simulink model "AprilTagHIL"  (R2024b)
settings: Solver=ode4  StartTime=0.0  StopTime=Tsim  FixedStep=0.005  RelTol=1e-3
values from neighbouring files (symbols this model uses):
  Caf = 20    [AprilTagHILSetup.m]
  Car = 20    [AprilTagHILSetup.m]
  circle_dir = 1    [AprilTagHILSetup.m]
  delta_corr_max_rad = deg2rad(8)    [AprilTagHILSetup.m]
  delta_max_rad = deg2rad(25)    [AprilTagHILSetup.m]
  delta_test_rad = deg2rad(14.6)    [AprilTagHILSetup.m]
  dist_psi_down_time_s = 10.0    (= 10)    [AprilTagHILSetup.m]
  dist_psi_step_amp_rad = deg2rad(10)    [AprilTagHILSetup.m]
  dist_psi_up_time_s = 9.0    (= 9)    [AprilTagHILSetup.m]
  dist_x_down_time_s = 6.0    (= 6)    [AprilTagHILSetup.m]
  dist_x_step_amp_m = 0.10    (= 0.1)    [AprilTagHILSetup.m]
  dist_x_up_time_s = 5.0    (= 5)    [AprilTagHILSetup.m]
  dist_y_down_time_s = 8.0    (= 8)    [AprilTagHILSetup.m]
  dist_y_up_time_s = 7.0    (= 7)    [AprilTagHILSetup.m]
  Jz = 0.015    [AprilTagHILSetup.m]
  K_psi = 0.8    [AprilTagHILSetup.m]
  K_r = 0.05    [AprilTagHILSetup.m]
  K_radius = 0.4    [AprilTagHILSetup.m]
  Kd_psi_pid = 0.0    (= 0)    [AprilTagHILSetup.m]
  Kd_radius_pid = 0.0    (= 0)    [AprilTagHILSetup.m]
  Ki_psi_pid = 0.0    (= 0)    [AprilTagHILSetup.m]
  Ki_radius_pid = 0.0    (= 0)    [AprilTagHILSetup.m]
  Kp_psi_pid = 1.0    (= 1)    [AprilTagHILSetup.m]
  Kp_radius_pid = 0.65    [AprilTagHILSetup.m]
  L = 0.26    [AprilTagHILSetup.m]
  lf = 0.13    [AprilTagHILSetup.m]
  lr = 0.13    [AprilTagHILSetup.m]
  m = 1.5    [AprilTagHILSetup.m]
  noise_psi_std_rad = deg2rad(0.5)    [AprilTagHILSetup.m]
  noise_x_std_m = 0.005    [AprilTagHILSetup.m]
  noise_y_std_m = 0.005    [AprilTagHILSetup.m]
  psi0_rad = pi/2 - deg2rad(45)    [AprilTagHILSetup.m]
  psi_offset_max_rad = deg2rad(18)    [AprilTagHILSetup.m]
  r0_radps = 0.0    (= 0)    [AprilTagHILSetup.m]
  R_ref = 1.0    (= 1)    [AprilTagHILSetup.m]
  Ts_vision = 0.05    [AprilTagHILSetup.m]
  Vx_const = 1.0    (= 1)    [AprilTagHILSetup.m]
  Vy0 = 0.0    (= 0)    [AprilTagHILSetup.m]
  X0 = 0.4    [AprilTagHILSetup.m]
  xc = 0.0    (= 0)    [AprilTagHILSetup.m]
  Y0 = 0.0    (= 0)    [AprilTagHILSetup.m]
  yc = 0.0    (= 0)    [AprilTagHILSetup.m]
libraries: slpidlib x2
settings Model: Creator=mateu  LastModifiedBy=mateu

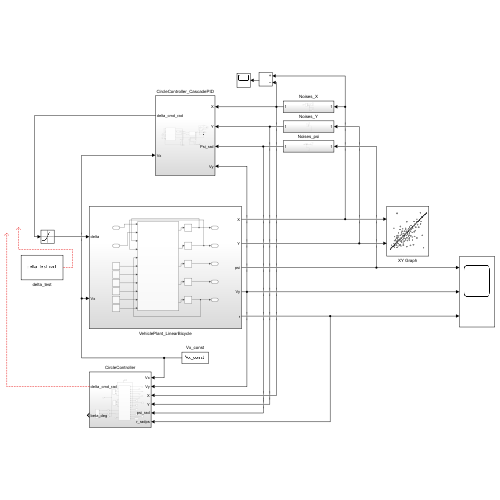
[thumbnail: Simulink's stored preview of the top-level diagram]
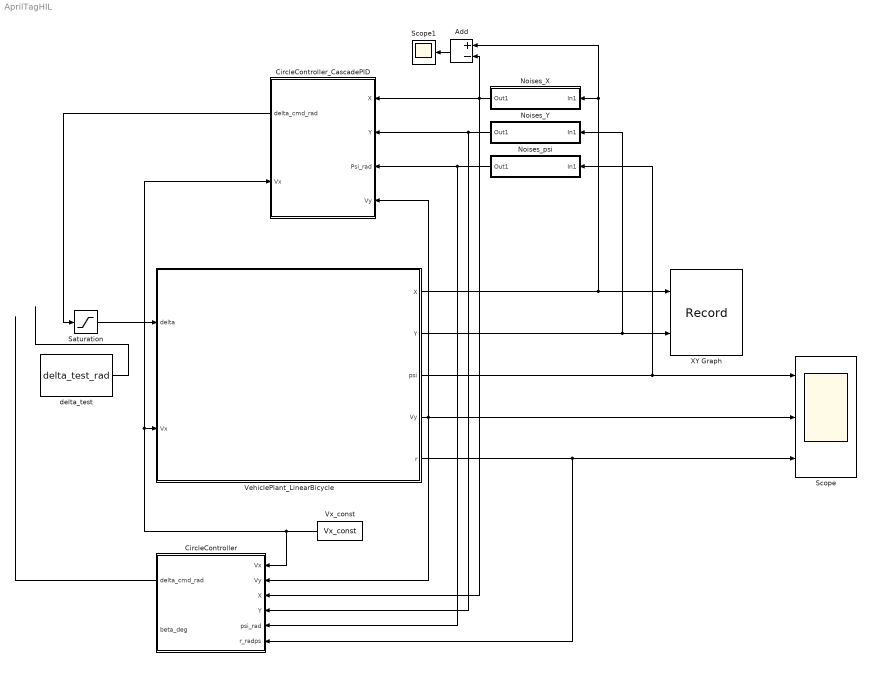
== system AprilTagHIL ==
  Add : Sum  Inputs=+-
  CircleController : Subsystem
  CircleController_CascadePID : Subsystem
      settings: PortSchema="{\"entries\":[{\"content\":{\"sides\":[{\"content\":{\"connectorIds\":[\"In1\",\"In2\",\"In3\",\"In4\"]},\"type\":\"ConnectorPlacement.EquallySpacedRectSide\",\"uuid\":\"4ebb86b3-f174-446a-9526-2905becb2528\"},{\"content\":{\"connectorIds\":[\"Out1\",\"In5\"],\"side\":\"RIGHT\"},\"type\":\"ConnectorPlacement.EquallySpacedRectSide\",\"uuid\":\"60998215-3f76-4645-a7df-e26e298f7453\"},{\"content\":{\"side\":\"TOP\"},\"type\":\"ConnectorPlacement.EquallySpacedRectSide\",\"uuid\":\"c14afc2e-0d09-4288-83d9-90a5a30cc5d5\"}]},\"type\":\"ConnectorPlacement.EquallySpacedConnector\",\"uuid\":\"bc3aa7c0-8848-4f28-b7fa-9a6d41e7c366\"}],\"packageUris\":[\"http://schema.mathworks.com/mf0/Connector/R2020b\"],\"version\":\"1.0\"}"
  Noises_X : Subsystem
  Noises_Y : Subsystem
  Noises_psi : Subsystem
  Saturation : Saturate  UpperLimit=delta_max_rad  LowerLimit=-delta_max_rad
  Scope : Scope  NumInputPorts=3
  Scope1 : Scope
  VehiclePlant_LinearBicycle : Subsystem
  Vx_const : Constant  Value=Vx_const
  XY Graph : Record  FileSettingsInternal="{\"entries\":[{\"content\":{\"excelSettings\":{\"content\":{},\"type\":\"Streamout.ExcelSettings\"}},\"type\":\"Streamout.FileSettingStorage\",\"uuid\":\"\"}],\"packageUris\":[\"http:\\/\\/schema.mathworks.com\\/mf0\\/streamout_blocks\\/R2020a\"],\"version\":\"1.0\"}"  Layout=[1 1]  SignalsInternal="{\"entries\":[{\"content\":{\"signals\":[{\"content\":{\"blockPath\":[],\"dimensions\":[1],\"domain\":\"\",\"lineColor\":\"#a2142f\",\"plots\":[ 1 ],\"port\":1,\"sid\":[\"\"],\"signalID\":1,\"signalName\":\"VehiclePlant_LinearBicycle:1\"},\"type\":\"RecordBlkView.Signal\",\"uuid\":\"\"},{\"content\":{\"blockPath\":[],\"dimensions\":[1],\"domain\":\"\",\"lineColor\":\"#139fff\",\"plots\":[ 1 ],\"port\":2,\"sid\":[\"\"],\"signalID\":2,\"signalName\":\"VehiclePlant_LinearBicycle:2\"},\"type\":\"RecordBlkView.Signal\",\"uuid\":\"\"}]},\"type\":\"RecordBlkView.InputSignals\",\"uuid\":\"\"}],\"packageUris\":[\"http:\\/\\/schema.mathworks.com\\/mf0\\/streamout_blocks\\/R2020a\"],\"version\":\"1.0\"}"  VisualizationBindings="{\"xyplotplugin\":{\"info\":[{\"series\":[{\"bindingParametersList\":[{\"parameter\":\"X-Axis\",\"signalID\":1,\"signalName\":\"VehiclePlant_LinearBicycle:1\"},{\"parameter\":\"Y-Axis\",\"signalID\":2,\"signalName\":\"VehiclePlant_LinearBicycle:2\"}],\"seriesID\":0}],\"subplotID\":1}]}}"  CompatibilityTag=XY
  delta_test : Constant  Value=delta_test_rad
  wires:
  Vx_const/1 -> CircleController/1(Vx), CircleController_CascadePID/5(Vx), VehiclePlant_LinearBicycle/2(Vx)
  Saturation/1 -> VehiclePlant_LinearBicycle/1(delta)
  VehiclePlant_LinearBicycle/1(X) -> XY Graph/1, Add/1, Noises_X/1(In1)
  VehiclePlant_LinearBicycle/4(Vy) -> CircleController_CascadePID/4(Vy), Scope/2, CircleController/2(Vy)
  VehiclePlant_LinearBicycle/5(r) -> Scope/3, CircleController/6(r_radps)
  VehiclePlant_LinearBicycle/3(psi) -> Noises_psi/1(In1), Scope/1
  VehiclePlant_LinearBicycle/2(Y) -> XY Graph/2, Noises_Y/1(In1)
  CircleController_CascadePID/1(delta_cmd_rad) -> Saturation/1
  Noises_Y/1(Out1) -> CircleController_CascadePID/2(Y), CircleController/4(Y)
  Noises_X/1(Out1) -> Add/2, CircleController_CascadePID/1(X), CircleController/3(X)
  Noises_psi/1(Out1) -> CircleController_CascadePID/3(Psi_rad), CircleController/5(psi_rad)
  Add/1 -> Scope1/1
  CircleController/1(delta_cmd_rad) -> ?
  delta_test/1 -> ?

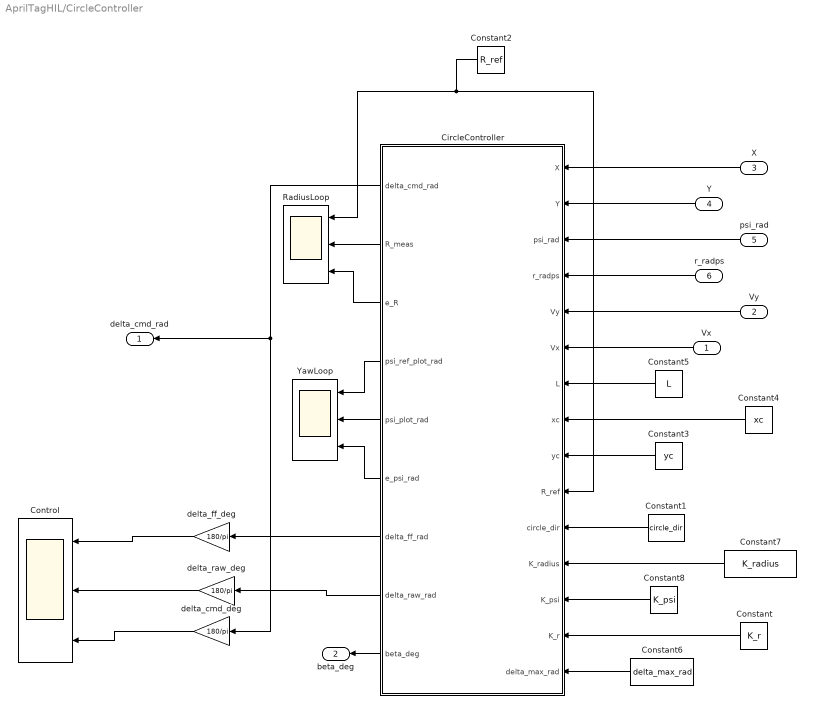
== system AprilTagHIL/CircleController ==
  Vx : Inport
  Vy : Inport  Port=2
  X : Inport  Port=3
  Y : Inport  Port=4
  psi_rad : Inport  Port=5
  r_radps : Inport  Port=6
  CircleController : MATLAB Function  TreatAsAtomicUnit=on
  Constant : Constant  Value=K_r
  Constant1 : Constant  Value=circle_dir
  Constant2 : Constant  Value=R_ref
  Constant3 : Constant  Value=yc
  Constant4 : Constant  Value=xc
  Constant5 : Constant  Value=L
  Constant6 : Constant  Value=delta_max_rad
  Constant7 : Constant  Value=K_radius
  Constant8 : Constant  Value=K_psi
  Control : Scope  NumInputPorts=3
  RadiusLoop : Scope  NumInputPorts=3
  YawLoop : Scope  NumInputPorts=3
  delta_cmd_deg : Gain  Gain=180/pi
  delta_ff_deg : Gain  Gain=180/pi
  delta_raw_deg : Gain  Gain=180/pi
  delta_cmd_rad : Outport
  beta_deg : Outport  Port=2
  wires:
  Vx/1 -> CircleController/6(Vx)
  CircleController/3(e_R) -> RadiusLoop/3
  CircleController/5(psi_plot_rad) -> YawLoop/2
  Constant1/1 -> CircleController/11(circle_dir)
  CircleController/7(delta_ff_rad) -> delta_ff_deg/1
  CircleController/9(beta_deg) -> beta_deg/1
  CircleController/4(psi_ref_plot_rad) -> YawLoop/1
  CircleController/6(e_psi_rad) -> YawLoop/3
  CircleController/8(delta_raw_rad) -> delta_raw_deg/1
  CircleController/2(R_meas) -> RadiusLoop/2
  CircleController/1(delta_cmd_rad) -> delta_cmd_deg/1, delta_cmd_rad/1
  Constant/1 -> CircleController/14(K_r)
  Constant4/1 -> CircleController/8(xc)
  X/1 -> CircleController/1(X)
  Constant3/1 -> CircleController/9(yc)
  Y/1 -> CircleController/2(Y)
  psi_rad/1 -> CircleController/3(psi_rad)
  r_radps/1 -> CircleController/4(r_radps)
  delta_raw_deg/1 -> Control/2
  Vy/1 -> CircleController/5(Vy)
  Constant5/1 -> CircleController/7(L)
  Constant7/1 -> CircleController/12(K_radius)
  Constant8/1 -> CircleController/13(K_psi)
  Constant6/1 -> CircleController/15(delta_max_rad)
  delta_ff_deg/1 -> Control/1
  delta_cmd_deg/1 -> Control/3
  Constant2/1 -> RadiusLoop/1, CircleController/10(R_ref)

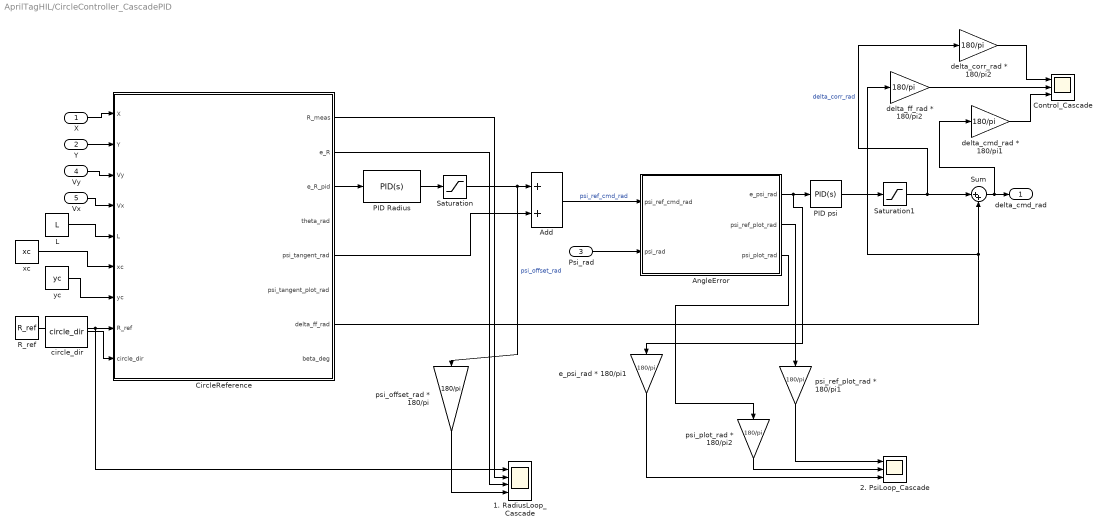
== system AprilTagHIL/CircleController_CascadePID ==
  X : Inport
  Y : Inport  Port=2
  Psi_rad : Inport  Port=3
  Vy : Inport  Port=4
  Vx : Inport  Port=5
  1. RadiusLoop_Cascade : Scope  NumInputPorts=4
  2. PsiLoop_Cascade : Scope  NumInputPorts=3
  Add : Sum
  AngleError : MATLAB Function  TreatAsAtomicUnit=on
  CircleReference : MATLAB Function  TreatAsAtomicUnit=on
  Control_Cascade : Scope  NumInputPorts=3
  L : Constant  Value=L
  PID Radius : slpidlib/PID Controller  Controller=PID  Form=Parallel  TimeDomain=Continuous-time  UseExternalTs=off  SampleTime=-1  IntegratorMethod=Forward Euler  FilterMethod=Forward Euler  ControllerParametersSource=internal  P=Kp_radius_pid  I=Ki_radius_pid  UseKiTs=off  D=Kd_radius_pid  UseExternalDerivativeSource=off  N=171.856773592637  UseFilter=on  TunerSelectOption=Transfer Function Based (PID Tuner App)  InitialConditionSource=internal  InitialConditionForIntegrator=0  InitialConditionForFilter=0  DifferentiatorICPrevScaledInput=0  ExternalReset=none  TrackingMode=off  Kt=1  LimitOutput=off  SatLimitsSource=internal  UpperSaturationLimit=inf  LowerSaturationLimit=-inf  LinearizeAsGain=on  AntiWindupMode=none  Kb=1  LimitIntegrator=off  UpperIntegratorSaturationLimit=inf  LowerIntegratorSaturationLimit=-inf  POutMin=[]  POutMax=[]  IOutMin=[]  IOutMax=[]  DOutMin=[]  DOutMax=[]  NOutMin=[]  NOutMax=[]  SumOutMin=[]  SumOutMax=[]  SaturationOutMin=[]  SaturationOutMax=[]  PParamMin=[]  PParamMax=[]  IParamMin=[]  IParamMax=[]  DParamMin=[]  DParamMax=[]  NParamMin=[]  NParamMax=[]  KbParamMin=[]  KbParamMax=[]  KtParamMin=[]  KtParamMax=[]  KbOutMin=[]  KbOutMax=[]  KtOutMin=[]  KtOutMax=[]  IntegratorOutMin=[]  IntegratorOutMax=[]  FilterOutMin=[]  FilterOutMax=[]  SumI1OutMin=[]  SumI1OutMax=[]  SumI2OutMin=[]  SumI2OutMax=[]  SumI3OutMin=[]  SumI3OutMax=[]  SumI4OutMin=[]  SumI4OutMax=[]  SumDOutMin=[]  SumDOutMax=[]  DifferentiatorOutMin=[]  DifferentiatorOutMax=[]  FilterDiffOutCoefMin=[]  FilterDiffOutCoefMax=[]  ReciprocalOutMin=[]  ReciprocalOutMax=[]  SumDenOutMin=[]  SumDenOutMax=[]  SumNumOutMin=[]  SumNumOutMax=[]  DivideOutMin=[]  DivideOutMax=[]  UdiffTsProdOutMin=[]  UdiffTsProdOutMax=[]  NTsProdOutMin=[]  NTsProdOutMax=[]  UintegralTsProdOutMin=[]  UintegralTsProdOutMax=[]  UngainTsProdOutMin=[]  UngainTsProdOutMax=[]  ClampingZeroOutDataTypeStr=Inherit: Inherit via back propagation  ClampingZeroOutMin=[]  ClampingZeroOutMax=[]  FilterDenConstantOutDataTypeStr=Inherit: Inherit via back propagation  FilterDenConstantOutMin=[]  FilterDenConstantOutMax=[]  PCopyOutDataTypeStr=Inherit: Inherit via back propagation  PCopyOutMin=[]  PCopyOutMax=[]  NCopyOutDataTypeStr=Inherit: Inherit via back propagation  NCopyOutMin=[]  NCopyOutMax=[]  IntegratorContinuousStateAttributes=''  IntegratorStateMustResolveToSignalObject=off  IntegratorRTWStateStorageClass=Auto  FilterContinuousStateAttributes=''  FilterStateMustResolveToSignalObject=off  FilterRTWStateStorageClass=Auto  ParallelPVariant=InternalParameters  IdealPVariant=Disabled  IVariant=InternalParameters  DVariant=InternalParameters  IntegratorVariant=Continuous  SatVariant=Disabled  AWVariant=Passthrough  PCopyVariant=Disabled  TRVariant=Disabled  FdbkBlocksVariant=Forward  IdealPFdbkVariant=Disabled  SatFdbkVariant=Disabled  DerivativeFilterVariant=ContFilter  NVariant=InternalParameters  NCopyVariant=Disabled  FilterICVariant=InternalICsFilter  IntegratorICVariant=InternalICs  ExternalResetVariant=Disabled  TRSumVariant=Passthrough  SumFdbkVariant=Disabled  SumVariant=Sum_PID  TsampFilterVariant=InternalTs  TsampNgainVariant=Passthrough  TsampIntegralVariant=Disabled_SignalSpec  ExternalSaturationOutDataTypeStr=Inherit: Same as second input  DerivativeSourceVariant=ErrorSignal  PreIntVariant=InternalPreInt
  PID psi : slpidlib/PID Controller  Controller=PID  Form=Parallel  TimeDomain=Continuous-time  UseExternalTs=off  SampleTime=-1  IntegratorMethod=Forward Euler  FilterMethod=Forward Euler  ControllerParametersSource=internal  P=Kp_psi_pid  I=Ki_psi_pid  UseKiTs=off  D=Kd_psi_pid  UseExternalDerivativeSource=off  N=184.215923888363  UseFilter=on  TunerSelectOption=Transfer Function Based (PID Tuner App)  InitialConditionSource=internal  InitialConditionForIntegrator=0  InitialConditionForFilter=0  DifferentiatorICPrevScaledInput=0  ExternalReset=none  TrackingMode=off  Kt=1  LimitOutput=off  SatLimitsSource=internal  UpperSaturationLimit=inf  LowerSaturationLimit=-inf  LinearizeAsGain=on  AntiWindupMode=none  Kb=1  LimitIntegrator=off  UpperIntegratorSaturationLimit=inf  LowerIntegratorSaturationLimit=-inf  POutMin=[]  POutMax=[]  IOutMin=[]  IOutMax=[]  DOutMin=[]  DOutMax=[]  NOutMin=[]  NOutMax=[]  SumOutMin=[]  SumOutMax=[]  SaturationOutMin=[]  SaturationOutMax=[]  PParamMin=[]  PParamMax=[]  IParamMin=[]  IParamMax=[]  DParamMin=[]  DParamMax=[]  NParamMin=[]  NParamMax=[]  KbParamMin=[]  KbParamMax=[]  KtParamMin=[]  KtParamMax=[]  KbOutMin=[]  KbOutMax=[]  KtOutMin=[]  KtOutMax=[]  IntegratorOutMin=[]  IntegratorOutMax=[]  FilterOutMin=[]  FilterOutMax=[]  SumI1OutMin=[]  SumI1OutMax=[]  SumI2OutMin=[]  SumI2OutMax=[]  SumI3OutMin=[]  SumI3OutMax=[]  SumI4OutMin=[]  SumI4OutMax=[]  SumDOutMin=[]  SumDOutMax=[]  DifferentiatorOutMin=[]  DifferentiatorOutMax=[]  FilterDiffOutCoefMin=[]  FilterDiffOutCoefMax=[]  ReciprocalOutMin=[]  ReciprocalOutMax=[]  SumDenOutMin=[]  SumDenOutMax=[]  SumNumOutMin=[]  SumNumOutMax=[]  DivideOutMin=[]  DivideOutMax=[]  UdiffTsProdOutMin=[]  UdiffTsProdOutMax=[]  NTsProdOutMin=[]  NTsProdOutMax=[]  UintegralTsProdOutMin=[]  UintegralTsProdOutMax=[]  UngainTsProdOutMin=[]  UngainTsProdOutMax=[]  ClampingZeroOutDataTypeStr=Inherit: Inherit via back propagation  ClampingZeroOutMin=[]  ClampingZeroOutMax=[]  FilterDenConstantOutDataTypeStr=Inherit: Inherit via back propagation  FilterDenConstantOutMin=[]  FilterDenConstantOutMax=[]  PCopyOutDataTypeStr=Inherit: Inherit via back propagation  PCopyOutMin=[]  PCopyOutMax=[]  NCopyOutDataTypeStr=Inherit: Inherit via back propagation  NCopyOutMin=[]  NCopyOutMax=[]  IntegratorContinuousStateAttributes=''  IntegratorStateMustResolveToSignalObject=off  IntegratorRTWStateStorageClass=Auto  FilterContinuousStateAttributes=''  FilterStateMustResolveToSignalObject=off  FilterRTWStateStorageClass=Auto  ParallelPVariant=InternalParameters  IdealPVariant=Disabled  IVariant=InternalParameters  DVariant=InternalParameters  IntegratorVariant=Continuous  SatVariant=Disabled  AWVariant=Passthrough  PCopyVariant=Disabled  TRVariant=Disabled  FdbkBlocksVariant=Forward  IdealPFdbkVariant=Disabled  SatFdbkVariant=Disabled  DerivativeFilterVariant=ContFilter  NVariant=InternalParameters  NCopyVariant=Disabled  FilterICVariant=InternalICsFilter  IntegratorICVariant=InternalICs  ExternalResetVariant=Disabled  TRSumVariant=Passthrough  SumFdbkVariant=Disabled  SumVariant=Sum_PID  TsampFilterVariant=InternalTs  TsampNgainVariant=Passthrough  TsampIntegralVariant=Disabled_SignalSpec  ExternalSaturationOutDataTypeStr=Inherit: Same as second input  DerivativeSourceVariant=ErrorSignal  PreIntVariant=InternalPreInt
  R_ref : Constant  Value=R_ref
  Saturation : Saturate  UpperLimit=psi_offset_max_rad  LowerLimit=-psi_offset_max_rad
  Saturation1 : Saturate  UpperLimit=delta_corr_max_rad  LowerLimit=-delta_corr_max_rad
  Sum : Sum  Inputs=|++
  circle_dir : Constant  Value=circle_dir
  delta_cmd_rad * 180/pi1 : Gain  Gain=180/pi
  delta_corr_rad * 180/pi2 : Gain  Gain=180/pi
  delta_ff_rad * 180/pi2 : Gain  Gain=180/pi
  e_psi_rad * 180/pi1 : Gain  Gain=180/pi
  psi_offset_rad * 180/pi : Gain  Gain=180/pi
  psi_plot_rad * 180/pi2 : Gain  Gain=180/pi
  psi_ref_plot_rad * 180/pi1 : Gain  Gain=180/pi
  xc : Constant  Value=xc
  yc : Constant  Value=yc
  delta_cmd_rad : Outport
  wires:
  X/1 -> CircleReference/1(X)
  Y/1 -> CircleReference/2(Y)
  Vy/1 -> CircleReference/3(Vy)
  Vx/1 -> CircleReference/4(Vx)
  yc/1 -> CircleReference/7(yc)
  R_ref/1 -> 1. RadiusLoop_Cascade/1, CircleReference/8(R_ref)
  circle_dir/1 -> CircleReference/9(circle_dir)
  L/1 -> CircleReference/5(L)
  xc/1 -> CircleReference/6(xc)
  CircleReference/3(e_R_pid) -> PID Radius/1
  PID Radius/1 -> Saturation/1
  Saturation/1 -> psi_offset_rad * 180/pi/1, Add/1  "psi_offset_rad"
  CircleReference/5(psi_tangent_rad) -> Add/2
  Add/1 -> AngleError/1(psi_ref_cmd_rad)  "psi_ref_cmd_rad"
  Psi_rad/1 -> AngleError/2(psi_rad)
  PID psi/1 -> Saturation1/1
  Saturation1/1 -> delta_corr_rad * 180/pi2/1, Sum/1  "delta_corr_rad"
  Sum/1 -> delta_cmd_rad * 180/pi1/1, delta_cmd_rad/1
  CircleReference/7(delta_ff_rad) -> delta_ff_rad * 180/pi2/1, Sum/2
  CircleReference/1(R_meas) -> 1. RadiusLoop_Cascade/2
  CircleReference/2(e_R) -> 1. RadiusLoop_Cascade/3
  psi_offset_rad * 180/pi/1 -> 1. RadiusLoop_Cascade/4
  AngleError/2(psi_ref_plot_rad) -> psi_ref_plot_rad * 180/pi1/1
  psi_ref_plot_rad * 180/pi1/1 -> 2. PsiLoop_Cascade/1
  psi_plot_rad * 180/pi2/1 -> 2. PsiLoop_Cascade/2
  e_psi_rad * 180/pi1/1 -> 2. PsiLoop_Cascade/3
  AngleError/3(psi_plot_rad) -> psi_plot_rad * 180/pi2/1
  delta_corr_rad * 180/pi2/1 -> Control_Cascade/1
  delta_ff_rad * 180/pi2/1 -> Control_Cascade/2
  delta_cmd_rad * 180/pi1/1 -> Control_Cascade/3
  AngleError/1(e_psi_rad) -> e_psi_rad * 180/pi1/1, PID psi/1

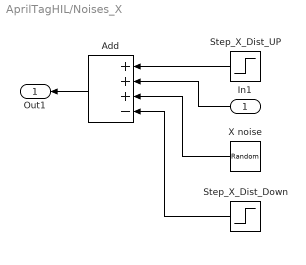
== system AprilTagHIL/Noises_X ==
  In1 : Inport
  Add : Sum  Inputs=+++-
  Step_X_Dist_Down : Step  Time=dist_x_down_time_s  After=dist_x_step_amp_m  SampleTime=0
  Step_X_Dist_UP : Step  Time=dist_x_up_time_s  After=dist_x_step_amp_m  SampleTime=0
  X noise : RandomNumber  Variance=noise_x_std_m^2  SampleTime=Ts_vision
  Out1 : Outport
  wires:
  In1/1 -> Add/2
  Add/1 -> Out1/1
  Step_X_Dist_Down/1 -> Add/4
  Step_X_Dist_UP/1 -> Add/1
  X noise/1 -> Add/3

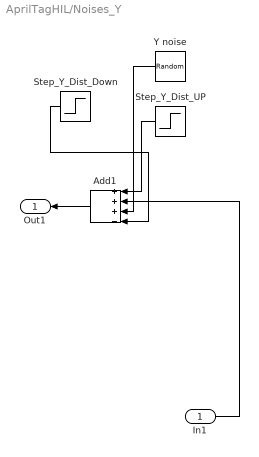
== system AprilTagHIL/Noises_Y ==
  In1 : Inport
  Add1 : Sum  Inputs=+++-
  Step_Y_Dist_Down : Step  Time=dist_y_down_time_s  After=dist_x_step_amp_m  SampleTime=0
  Step_Y_Dist_UP : Step  Time=dist_y_up_time_s  After=dist_x_step_amp_m  SampleTime=0
  Y noise : RandomNumber  Variance=noise_y_std_m^2  SampleTime=Ts_vision
  Out1 : Outport
  wires:
  Y noise/1 -> Add1/3
  Add1/1 -> Out1/1
  Step_Y_Dist_UP/1 -> Add1/1
  In1/1 -> Add1/2
  Step_Y_Dist_Down/1 -> Add1/4

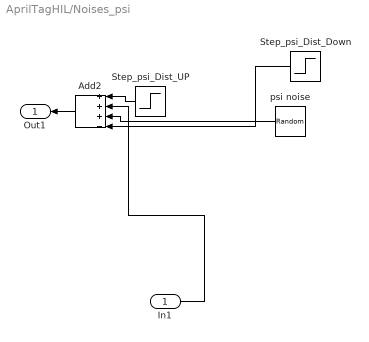
== system AprilTagHIL/Noises_psi ==
  In1 : Inport
  Add2 : Sum  Inputs=+++-
  Step_psi_Dist_Down : Step  Time=dist_psi_down_time_s  After=dist_psi_step_amp_rad  SampleTime=0
  Step_psi_Dist_UP : Step  Time=dist_psi_up_time_s  After=dist_psi_step_amp_rad  SampleTime=0
  psi noise : RandomNumber  Variance=noise_psi_std_rad^2  SampleTime=Ts_vision
  Out1 : Outport
  wires:
  psi noise/1 -> Add2/3
  In1/1 -> Add2/2
  Step_psi_Dist_UP/1 -> Add2/1
  Step_psi_Dist_Down/1 -> Add2/4
  Add2/1 -> Out1/1

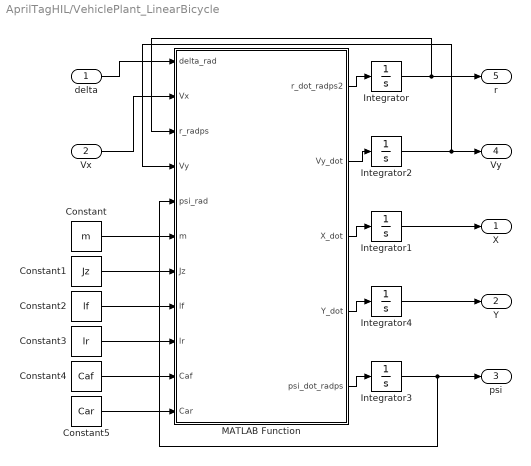
== system AprilTagHIL/VehiclePlant_LinearBicycle ==
  delta : Inport
  Vx : Inport  Port=2
  Constant : Constant  Value=m
  Constant1 : Constant  Value=Jz
  Constant2 : Constant  Value=lf
  Constant3 : Constant  Value=lr
  Constant4 : Constant  Value=Caf
  Constant5 : Constant  Value=Car
  Integrator : Integrator  InitialCondition=r0_radps
  Integrator1 : Integrator  InitialCondition=X0
  Integrator2 : Integrator  InitialCondition=Vy0
  Integrator3 : Integrator  InitialCondition=psi0_rad
  Integrator4 : Integrator  InitialCondition=Y0
  MATLAB Function : MATLAB Function  TreatAsAtomicUnit=on
  X : Outport
  Y : Outport  Port=2
  psi : Outport  Port=3
  Vy : Outport  Port=4
  r : Outport  Port=5
  wires:
  MATLAB Function/4(Y_dot) -> Integrator4/1
  MATLAB Function/1(r_dot_radps2) -> Integrator/1
  MATLAB Function/2(Vy_dot) -> Integrator2/1
  MATLAB Function/5(psi_dot_radps) -> Integrator3/1
  MATLAB Function/3(X_dot) -> Integrator1/1
  Integrator3/1 -> MATLAB Function/5(psi_rad), psi/1
  Integrator/1 -> MATLAB Function/3(r_radps), r/1
  Integrator1/1 -> X/1
  Integrator2/1 -> Vy/1, MATLAB Function/4(Vy)
  Vx/1 -> MATLAB Function/2(Vx)
  delta/1 -> MATLAB Function/1(delta_rad)
  Integrator4/1 -> Y/1
  Constant/1 -> MATLAB Function/6(m)
  Constant1/1 -> MATLAB Function/7(Jz)
  Constant2/1 -> MATLAB Function/8(lf)
  Constant3/1 -> MATLAB Function/9(lr)
  Constant4/1 -> MATLAB Function/10(Caf)
  Constant5/1 -> MATLAB Function/11(Car)

== matlab function AprilTagHIL/CircleController_CascadePID/AngleError ==
  data: psi_ref_cmd_rad input; e_psi_rad output; psi_rad input; psi_ref_plot_rad output; psi_plot_rad output
function [e_psi_rad, psi_ref_plot_rad, psi_plot_rad] = AngleError(psi_ref_cmd_rad, psi_rad)
% AngleError
%
% Liczy uchyb orientacji:
%
%   e_psi = psi_ref_cmd - psi
%
% z zawinięciem do -pi..pi, żeby uniknąć skoku np. 179 deg -> -179 deg.
%
% PID nie musi mieć wyjścia w tej samej jednostce co wejście.
% Tutaj:
%
%   e_psi_rad -> PID_Psi -> delta_corr_rad
%
% czyli uchyb orientacji [rad] jest przeliczany przez wzmocnienia PID
% na korektę skrętu kół [rad].
%
% To jest analogiczne do:
%
%   uchyb temperatury [degC] -> PID -> moc grzałki [%]

e_psi_rad = atan2(sin(psi_ref_cmd_rad - psi_rad), cos(psi_ref_cmd_rad - psi_rad));

psi_ref_plot_rad = atan2(sin(psi_ref_cmd_rad), cos(psi_ref_cmd_rad));
psi_plot_rad     = atan2(sin(psi_rad),         cos(psi_rad));

end

== matlab function AprilTagHIL/CircleController/CircleController ==
  data: X input; delta_cmd_rad output; Y input; psi_rad input; r_radps input; Vy input; Vx input; R_meas output; e_R output; psi_ref_plot_rad output; psi_plot_rad output; e_psi_rad output; delta_ff_rad output; delta_raw_rad output; beta_deg output; L input; xc input; yc input; R_ref input; circle_dir input; K_radius input; K_psi input; K_r input; delta_max_rad input
function [delta_cmd_rad, R_meas, e_R, psi_ref_plot_rad, psi_plot_rad, e_psi_rad, delta_ff_rad, delta_raw_rad, beta_deg] = CircleController(X, Y, psi_rad, r_radps, Vy, Vx, L, xc, yc, R_ref, circle_dir, K_radius, K_psi, K_r, delta_max_rad)
% CircleController
%
% Konwencja:
% psi   - orientacja pojazdu / yaw [rad]
% r     - yaw rate = dpsi/dt [rad/s]
% delta - kąt skrętu kół [rad]
% beta  - kąt poślizgu bocznego [rad]
% theta - kąt położenia pojazdu względem środka okręgu [rad]
%
% UWAGA:
% theta_rad NIE jest orientacją pojazdu.
% theta_rad mówi tylko, gdzie pojazd znajduje się na okręgu.

% =========================
% Pozycja względem środka okręgu
% =========================

dx = X - xc;
dy = Y - yc;

% =========================
% Pętla promienia
% =========================

% Wartość mierzona promienia
R_meas = sqrt(dx*dx + dy*dy);

% Uchyb promienia: wartość zadana - wartość mierzona
e_R = R_ref - R_meas;

% =========================
% Kąt położenia na okręgu
% =========================

% theta_rad mówi, gdzie auto jest na okręgu.
% To NIE jest yaw.
theta_rad = atan2(dy, dx);

% =========================
% Pętla orientacji psi
% =========================

% Zadana orientacja pojazdu: styczna do okręgu
psi_ref_rad = theta_rad + circle_dir*pi/2;

% Wersje do wykresów, zawinięte do -pi..pi
psi_ref_plot_rad = atan2(sin(psi_ref_rad), cos(psi_ref_rad));
psi_plot_rad     = atan2(sin(psi_rad),     cos(psi_rad));

% Uchyb orientacji:
% e_psi = psi_ref - psi
e_psi_rad = atan2(sin(psi_ref_rad - psi_rad), cos(psi_ref_rad - psi_rad));

% =========================
% Feedforward skrętu
% =========================

% Geometria modelu rowerowego:
% delta = atan(L / R)
delta_ff_rad = circle_dir * atan(L / R_ref);

% =========================
% Korekcje regulatora
% =========================

% Korekta od promienia.
% Dla CCW:
% e_R < 0 oznacza R_meas > R_ref, czyli auto jest za daleko od środka.
% Wtedy człon (-K_radius * e_R) zwiększa skręt do środka.
delta_radius_corr_rad = circle_dir * (-K_radius * e_R);

% Korekta od orientacji psi
delta_psi_corr_rad = K_psi * e_psi_rad;

% Tłumienie yaw rate r
delta_r_damping_rad = -K_r * r_radps;

% Skręt przed saturacją
delta_raw_rad = delta_ff_rad ...
              + delta_radius_corr_rad ...
              + delta_psi_corr_rad ...
              + delta_r_damping_rad;

% =========================
% Saturacja skrętu
% =========================

if delta_raw_rad > delta_max_rad
    delta_cmd_rad = delta_max_rad;
elseif delta_raw_rad < -delta_max_rad
    delta_cmd_rad = -delta_max_rad;
else
    delta_cmd_rad = delta_raw_rad;
end

% =========================
% Diagnostyka kąta poślizgu
% =========================

beta_rad = atan2(Vy, Vx);
beta_deg = beta_rad * 180/pi;

end

== matlab function AprilTagHIL/VehiclePlant_LinearBicycle/MATLAB Function ==
  data: delta_rad input; r_dot_radps2 output; Vx input; r_radps input; Vy input; psi_rad input; Vy_dot output; X_dot output; Y_dot output; psi_dot_radps output; m input; Jz input; lf input; lr input; Caf input; Car input
function [r_dot_radps2, Vy_dot, X_dot, Y_dot, psi_dot_radps] = BicycleDynamics(delta_rad, Vx, r_radps, Vy, psi_rad, m, Jz, lf, lr, Caf, Car)
% BicycleDynamics
%
% Konwencja:
% psi   - orientacja pojazdu / yaw [rad]
% r     - yaw rate = dpsi/dt [rad/s]
% delta - kąt skrętu kół [rad]
% Vy    - prędkość boczna w układzie pojazdu [m/s]
% Vx    - prędkość wzdłużna w układzie pojazdu [m/s]

% =========================
% Zabezpieczenia numeryczne
% =========================

Vx_min_local = 0.1;

if Vx < Vx_min_local
    Vx_eff = Vx_min_local;
else
    Vx_eff = Vx;
end

if Jz <= 0
    Jz_eff = 0.01;
else
    Jz_eff = Jz;
end

% =========================
% Kąty poślizgu opon
% =========================

alpha_f = atan((Vy + lf*r_radps) / Vx_eff) - delta_rad;
alpha_r = atan((Vy - lr*r_radps) / Vx_eff);

% =========================
% Liniowy model sił bocznych
% =========================

Fy_f = -Caf * alpha_f;
Fy_r = -Car * alpha_r;

% =========================
% Dynamika yaw i prędkości bocznej
% =========================

r_dot_radps2 = (lf * Fy_f * cos(delta_rad) - lr * Fy_r) / Jz_eff;

Vy_dot = (Fy_f * cos(delta_rad) + Fy_r) / m - r_radps * Vx;

% =========================
% Kinematyka globalna
% =========================

psi_dot_radps = r_radps;

X_dot = Vx * cos(psi_rad) - Vy * sin(psi_rad);
Y_dot = Vx * sin(psi_rad) + Vy * cos(psi_rad);

end

== matlab function AprilTagHIL/CircleController_CascadePID/CircleReference ==
  data: X input; R_meas output; Y input; Vy input; Vx input; L input; xc input; yc input; R_ref input; circle_dir input; e_R output; e_R_pid output; theta_rad output; psi_tangent_rad output; psi_tangent_plot_rad output; delta_ff_rad output; beta_deg output
function [R_meas, e_R, e_R_pid, theta_rad, psi_tangent_rad, psi_tangent_plot_rad, delta_ff_rad, beta_deg] = CircleReference(X, Y, Vy, Vx, L, xc, yc, R_ref, circle_dir)
% CircleReference
%
% Blok geometrii okręgu.
%
% Konwencja:
% theta - kąt położenia pojazdu względem środka okręgu, NIE yaw
% psi   - orientacja pojazdu / yaw
% delta - kąt skrętu kół
%
% Łańcuch fizyczny:
%
%   delta -> r -> psi -> X,Y -> R_meas
%
% delta nie zmienia promienia bezpośrednio. Najpierw zmienia yaw rate r,
% potem orientację psi, potem kierunek ruchu, a dopiero potem pozycję X,Y
% i promień R_meas.
%
% Dlatego w kaskadzie:
%
%   PID promienia: e_R -> psi_offset
%   PID psi:       e_psi -> delta_corr

dx = X - xc;
dy = Y - yc;

% Mierzony promień od środka okręgu
R_meas = sqrt(dx*dx + dy*dy);

% Klasyczny uchyb do wykresów:
% e_R > 0 -> auto jest za blisko środka
% e_R < 0 -> auto jest za daleko od środka
e_R = R_ref - R_meas;

% Sygnał na PID promienia.
% Znak uwzględnia kierunek jazdy po okręgu.
e_R_pid = -circle_dir * e_R;

% Kąt położenia na okręgu
% To NIE jest orientacja auta.
theta_rad = atan2(dy, dx);

% Kierunek styczny do okręgu
psi_tangent_rad = theta_rad + circle_dir*pi/2;

% Do wykresu zawijamy do -pi..pi
psi_tangent_plot_rad = atan2(sin(psi_tangent_rad), cos(psi_tangent_rad));

% Feedforward skrętu wynikający z geometrii modelu rowerowego
% delta_ff = atan(L/R)
delta_ff_rad = circle_dir * atan(L / R_ref);

% Diagnostyka poślizgu bocznego
beta_rad = atan2(Vy, Vx);
beta_deg = beta_rad * 180/pi;

end
